simulink model "fxpdemo_fix2fix"  (Simulink 5.0)
settings: Solver=FixedStepDiscrete  SolverMode=SingleTasking  StartTime=0.0  StopTime=0.9985  FixedStep=0.001  RelTol=1e-3  AbsTol=1e-6
libraries: fixpt_lib_4 x4, fixpt_lib_3p1 x1
settings Model: RequirementInfo=9  CovMetricSettings=d  MinMaxOverflowLogging=MinMaxAndOverflow  Creator=andyb  LastModifiedBy=andyb  ExtModeTrigMode=oneshot  ExtModeArmWhenConnect=off  ExtModeAutoUpdateStatusClock=off  LimitDataPoints=off  IntegerOverflowMsg=none  ParameterDowncastMsg=warning  ParameterOverflowMsg=warning  ParameterPrecisionLossMsg=none  BooleanDataType=off  RTWOptions="-aRollThreshold=5 -aShowEliminatedStatements=1 -aRTWVerbose=1 -aLocalBlockOutputs=1 -aInlineInvariantSignals=1 -aLogVarNameModifier=\"rt_\""

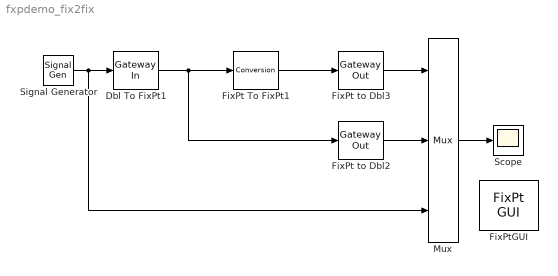
== system fxpdemo_fix2fix ==
  Dbl To FixPt1 : fixpt_lib_4/Data Type/Gateway In  InRealWorld=Real World Value  OutputDataTypeScalingMode=Specify via dialog  OutDataType=sfix(32)  OutScaling=2^-2  RndMeth=Nearest  DoSatur=on
  FixPt To FixPt1 : fixpt_lib_4/Data Type/Conversion  ConvertRealWorld=Real World Value  OutputDataTypeScalingMode=Specify via dialog  OutDataType=ufix(8)  OutScaling=2^-1  DoSatur=on
  FixPt to Dbl2 : fixpt_lib_4/Data Type/Gateway Out  OutRealWorld=Real World Value  OutBuiltInType=double  DoSatur=off
  FixPt to Dbl3 : fixpt_lib_4/Data Type/Gateway Out  OutRealWorld=Real World Value  OutBuiltInType=double  DoSatur=off
  FixPtGUI : fixpt_lib_3p1/FixPt GUI
  Mux : Mux  Inputs=3
  Scope : Scope
      settings: TickLabels=on
  Signal Generator : SignalGenerator  WaveForm=sawtooth  Amplitude=5
  wires:
  Signal Generator/1 -> Dbl To FixPt1/1, Mux/3
  FixPt To FixPt1/1 -> FixPt to Dbl3/1
  FixPt to Dbl2/1 -> Mux/2
  FixPt to Dbl3/1 -> Mux/1
  Dbl To FixPt1/1 -> FixPt To FixPt1/1, FixPt to Dbl2/1
  Mux/1 -> Scope/1
